simulink model "SetWheelVelocity"  (R2017b)
settings: Solver=VariableStepAuto  StartTime=0.0  StopTime=10.0  RelTol=1e-3
libraries: realtime_pacer_lib x1
settings Model: Creator=wafflefries  LastModifiedBy=wafflefries

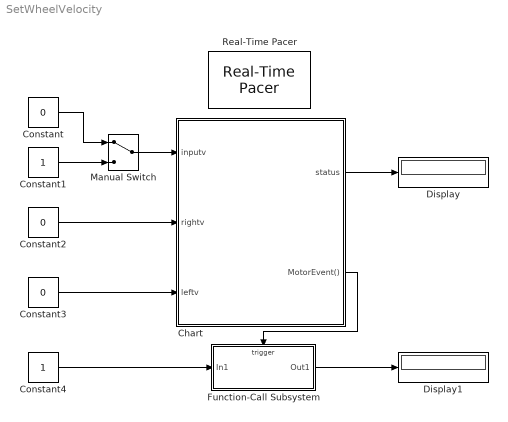
== system SetWheelVelocity ==
  Chart : Stateflow chart  TreatAsAtomicUnit=on
  Constant : Constant  Value=0
  Constant1 : Constant
  Constant2 : Constant  Value=0
  Constant3 : Constant  Value=0
  Constant4 : Constant
  Display : Display
  Display1 : Display
  Function-Call Subsystem : Subsystem  TreatAsAtomicUnit=on
  Manual Switch : ManualSwitch
  Real-Time Pacer : realtime_pacer_lib/Real-Time Pacer  simTimePerRealTime=0.5
  wires:
  Constant2/1 -> Chart/2(rightv)
  Constant3/1 -> Chart/3(leftv)
  Manual Switch/1 -> Chart/1(inputv)
  Constant/1 -> Manual Switch/1
  Constant1/1 -> Manual Switch/2
  Chart/1(status) -> Display/1
  Chart/2(MotorEvent()) -> Function-Call Subsystem/Trigger
  Constant4/1 -> Function-Call Subsystem/1(In1)
  Function-Call Subsystem/1(Out1) -> Display1/1

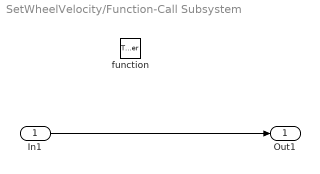
== system SetWheelVelocity/Function-Call Subsystem ==
  In1 : Inport
  function : TriggerPort  TriggerType=function-call  VariantControl=Variant
  Out1 : Outport
  wires:
  In1/1 -> Out1/1

== stateflow chart SetWheelVelocity/Chart ==
  state NOOP
    entry:
    status = 0;
  state START
    entry:
    coder.extrinsic('SetWheelVelRoomba')
    SetWheelVelRoomba(so, rightv, leftv)
    MotorEvent
    status = 1;
  state RESET
    entry:
  (default) -> NOOP : {
      | coder.extrinsic('RoombaWiFiInit')
      | so = RoombaWiFiInit(' ', 'full')
      | }
  RESET -> NOOP
  NOOP -> START : [inputv == 1]
  START -> RESET : [inputv == 0]
  data: inputv input; rightv input; leftv input; status output; so local
  events: MotorEvent output FUNCTION_CALL_EVENT
